simulink model "CM13_2024a_MachE_for_UA_HIL"  (R2024a)
settings: Solver=ode1  StartTime=0.0  StopTime=Inf  FixedStep=0.001  RelTol=1e-3  EnableMultiTasking=on
PreLoadFcn:
  | % if ~length(which('cmcmd')), cmenv; end
PostLoadFcn:
  | if any(exist('dsrtsu_mdlpostloadfcn', 'file') ~= 0), dsrtsu_mdlpostloadfcn('Execute', bdroot); end
InitFcn:
  | , if any(exist('rtifpga_mdlclblib', 'file') ~= 0), rtifpga_mdlclblib('Init', bdroot); end,
  | , if any(exist('dsmpb_private', 'file') ~= 0), dsmpb_private('dsmpb_mdlclblib', 'Init', bdroot); end,
values from neighbouring files (symbols this model uses):
  CoastDown =     [Run_Simulink.mat]
  limitedMCT =     [Run_Simulink.mat]
  MCT =     [Run_Simulink.mat]
  pMCT =     [Run_Simulink.mat]
  RealSimPara =     [Run_Simulink.mat]
  Ref_speed = [13 13.007895099 13.015778396 13.023649891 13.031509584 13.039357475 13.047193564 13.055017851 13.062830336 13.070631019 13.0784199 13.086196979 ... (2669 elements, 2669x1)]    [Ref_speed_and_time.mat]
  Ref_time = [0 0.01 0.02 0.03 0.04 0.05 0.06 0.07 0.08 0.09 0.1 0.11 ... (2669 elements, 2669x1)]    [Ref_speed_and_time.mat]
  US06 =     [Run_Simulink.mat]
undefined symbols (not defined in the file or in its folder): AccelCmd, ActTqLF_Nm_, ActTqLR_Nm_, ActTqRF_Nm_, ActTqRR_Nm_, BattChargeLimitMaxPwr, BattChargeLimitSocBpts, BattChargeLimitTbl, BattChrgCapcty, BattDischargeLimitSocBpts, BattDischargeLimitTbl, BattDischargeMaxPwr, BattNumCellsParallel, BattNumCellsSeries, BattOpenVoltCapBpts, BattOpenVoltTbl, BattResistSocBpts, BattResistTbl, BattResistTempBpts, BrakeMaxPrs, BrakeMaxTrq, ChassisDistCg2FrontAxle, ChassisDistCg2RearAxle, ChassisVehMass, CltchCmd, DecelCmd, DiffRatio, DiscIntNeverNeededParam, EnvGravCnst, EnvPrs, EnvTemp, FuelSpecificGrav, GearCmd, h, InitStates, lgSw, MtrEffSpdBpts, MtrEffTbl, MtrEffTrqBpts, MtrPwrMax, MtrTrqMax, planned_speed, planned_time, ref_speed, ref_time, rticanmm_blockfcn, rticanmm_initfcn, SteeringCmd, SupvsryCtrlRegenBrkCutOffTbl, SupvsryCtrlRegenSpdBpts, TestScnrioCycleNum, VEH
libraries: simulink x264, VSIGenLib x262, etargetslib x201, dsmpblib x161, CarMaker4SL x142, rtimmsu_dsrtlib x32, vehdynlibtire x24, autolibshared x19, vehdynlibsuspension x14, vehdynlibtirecommon x14, autolibutils x10, VsrLibWheel x8
(part 19 of 48)

== system CM13_2024a_MachE_for_UA_HIL/Vehicle Under Test3/Vehicle/Rototest and ORNL Interface/DummyPT ==
  WhlSpeedIn : Inport
  APPToTorque : Lookup_n-D  NumberOfTableDimensions=1  BreakpointsForDimension1=[0 100]  Table=[0 184]  InternalRulePriority=Speed  RndMeth=Simplest
  APPToTorque1 : Lookup_n-D  NumberOfTableDimensions=1  BreakpointsForDimension1=[0 100]  Table=[0 184]  InternalRulePriority=Speed  RndMeth=Simplest
  APP_pct : Constant  Value=0
  BPP_pct : Constant  Value=0
  FDR : Gain  Gain=3.18
  Flip : Gain  Gain=-1
  Gear : Product
  Memory : Memory
  NissanTrans : Lookup_n-D  NumberOfTableDimensions=1  BreakpointsForDimension1=[0 5 10 15 25 34 45 55]  Table=[5.25 3.03 1.95 1.46 1.22 1.00 0.81 0.67]  ExtrapMethod=Clip  InternalRulePriority=Speed  RndMeth=Simplest
  Sum : Sum  Inputs=++|
  WheelRadius : Gain  Gain=0.3235
  kph2mph : Gain  Gain=0.621
  mps2kph : Gain  Gain=3.6
  WheelTorqueOut : Outport
  wires:
  kph2mph/1 -> NissanTrans/1  "Speed_mph"
  APPToTorque/1 -> Sum/1  "APPTorque"
  mps2kph/1 -> kph2mph/1  "Speed_kph"
  BPP_pct/1 -> APPToTorque1/1
  NissanTrans/1 -> Gear/2  "Gear"
  Gear/1 -> FDR/1  "TransTorqueOut"
  APPToTorque1/1 -> Flip/1
  Flip/1 -> Sum/2  "BPPTorque"
  APP_pct/1 -> APPToTorque/1
  Sum/1 -> Gear/1  "TorqueTotal"
  WheelRadius/1 -> mps2kph/1  "Speed_mps"
  FDR/1 -> Memory/1  "WheelTorqueOut"
  WhlSpeedIn/1 -> WheelRadius/1
  Memory/1 -> WheelTorqueOut/1

== system CM13_2024a_MachE_for_UA_HIL/Vehicle Under Test3/Vehicle/Rototest and ORNL Interface/Format CM Powertrain Signals ==
  note: Can Bypass with my own brake model
  BrakingTorques : Inport
  RotoWheelSpd : Inport  Port=2
  AxlTrq : Inport  Port=3
  MaxRegen : Inport  Port=4
  Bus Creator1 : BusCreator  Inputs=42
  Bus Selector2 : BusSelector  OutputSignals=Brake IF Trq_WB FL,Brake IF Trq_WB FR,Brake IF Trq_WB RL,Brake IF Trq_WB RR
  BusCreator2 : BusCreator  Inputs=42
  Demux : Demux
  Demux1 : Demux  Outputs=42
      settings: DisplayOption=none
  Demux2 : Demux
  Discrete-Time Integrator{4..7} (4 alike) : DiscreteIntegrator  IntegratorMethod=Integration: Backward Euler  SampleTime=0.001  ICPrevOutput=DiscIntNeverNeededParam  ICPrevScaledInput=DiscIntNeverNeededParam
  Gain{5..8} (4 alike) : Gain  Gain=-1
  Ground{2..5} (4 alike) : Ground
  Ignition : Constant
  Memory{1..4} (4 alike) : Memory
  Operation Error : Constant  Value=4
  Operation State Driving : Constant  Value=4
  Product{1..4} (4 alike) : Product  RndMeth=Zero
  Saturation{1..4} (4 alike) : Saturate  UpperLimit=1  LowerLimit=-1
  Zero{1..5} (5 alike) : Constant  Value=0
  PowerTrainOutIdeal : Outport
  wires:
  Saturation4/1 -> Product4/2
  Demux1/3 -> BusCreator2/3  "PT IF OperationError"
  Demux1/2 -> BusCreator2/2  "PT IF OperationState"
  Demux1/40 -> BusCreator2/40  "PT IF WRR Trq_Supp2WC"
  Demux1/9 -> BusCreator2/9  "PT IF Trq_Supp2Bdy1B x"
  Discrete-Time Integrator6/1 -> Bus Creator1/29  "PT WRL rot"
  Demux1/1 -> BusCreator2/1  "PT IF Ignition"
  MaxRegen/1 -> Bus Creator1/28, Bus Creator1/21
  BusCreator2/1 -> PowerTrainOutIdeal/1
  Operation State Driving/1 -> Bus Creator1/2
  Gain8/1 -> Bus Creator1/38
  Demux1/16 -> BusCreator2/16  "PT IF WFL rotv"
  Demux1/21 -> BusCreator2/21  "PT IF WFL Trq_BrakeReg_max"
  Ground2/1 -> Bus Creator1/7
  Demux1/23 -> BusCreator2/23  "PT IF WFR rotv"
  Demux1/14 -> BusCreator2/14  "PT IF DL_iDiff_mean"
  Demux1/4 -> BusCreator2/4  "PT IF GearNo"
  Demux1/17 -> BusCreator2/17  "PT IF WFL Trq_B2W"
  Product3/1 -> Gain5/1
  Demux1/5 -> BusCreator2/5  "PT IF Engine_rotv"
  Demux1/11 -> BusCreator2/11  "PT IF Trq_Supp2Bdy1B z"
  Demux1/12 -> BusCreator2/12  "PT IF Trq_Supp2BdyEng x"
  Demux1/7 -> BusCreator2/7  "PT IF Trq_Supp2Bdy1 y"
  Discrete-Time Integrator5/1 -> Bus Creator1/22  "PT WFR rot"
  Demux1/42 -> BusCreator2/42  "PT IF WRR Trq_BrakeReg_max"
  Gain5/1 -> Bus Creator1/17
  Demux1/18 -> BusCreator2/18  "PT IF WFL Trq_Drive"
  Demux1/8 -> BusCreator2/8  "PT IF Trq_Supp2Bdy1 z"
  Demux1/38 -> BusCreator2/38  "PT IF WRR Trq_B2W"
  Memory4/1 -> Saturation4/1
  Demux1/10 -> BusCreator2/10  "PT IF Trq_Supp2Bdy1B y"
  Demux1/27 -> BusCreator2/27  "PT IF WFR Trq_BrakeReg"
  Demux1/24 -> BusCreator2/24  "PT IF WFR Trq_B2W"
  Demux1/25 -> BusCreator2/25  "PT IF WFR Trq_Drive"
  Demux1/26 -> BusCreator2/26  "PT IF WFR Trq_Supp2WC"
  Demux1/13 -> BusCreator2/13  "PT IF Trq_Supp2BdyEng y"
  Demux1/15 -> BusCreator2/15  "PT IF WFL rot"
  Bus Selector2/2 -> Product1/1  "<Brake IF Trq_WB FR>"
  Memory3/1 -> Saturation3/1
  Demux1/19 -> BusCreator2/19  "PT IF WFL Trq_Supp2WC"
  Demux1/22 -> BusCreator2/22  "PT IF WFR rot"
  Demux1/29 -> BusCreator2/29  "PT IF WRL rot"
  Demux1/33 -> BusCreator2/33  "PT IF WRL Trq_Supp2WC"
  Demux1/30 -> BusCreator2/30  "PT IF WRL rotv"
  Demux1/28 -> BusCreator2/28  "PT IF WFR Trq_BrakeReg_max"
  Demux1/35 -> BusCreator2/35  "PT IF WRL Trq_BrakeReg_max"
  Demux1/39 -> BusCreator2/39  "PT IF WRR Trq_Drive"
  Zero4/1 -> Bus Creator1/33, Bus Creator1/34, Bus Creator1/35
  Demux1/34 -> BusCreator2/34  "PT IF WRL Trq_BrakeReg"
  Demux1/37 -> BusCreator2/37  "PT IF WRR rotv"
  Demux1/31 -> BusCreator2/31  "PT IF WRL Trq_B2W"
  Demux1/32 -> BusCreator2/32  "PT IF WRL Trq_Drive"
  Demux1/36 -> BusCreator2/36  "PT IF WRR rot"
  Zero3/1 -> Bus Creator1/26, Bus Creator1/27
  Demux/4 -> Memory4/1, Discrete-Time Integrator7/1, Bus Creator1/37  "rotv RR"
  Zero2/1 -> Bus Creator1/19, Bus Creator1/20
  Zero1/1 -> Bus Creator1/5, Bus Creator1/4, Bus Creator1/12, Bus Creator1/14, Bus Creator1/13, Bus Creator1/11, Bus Creator1/10, Bus Creator1/9, Bus Creator1/8
  Demux1/20 -> BusCreator2/20  "PT IF WFL Trq_BrakeReg"
  Product2/1 -> Gain7/1
  Discrete-Time Integrator4/1 -> Bus Creator1/15  "PT WFL rot"
  Demux/2 -> Memory1/1, Discrete-Time Integrator5/1, Bus Creator1/23  "rotv FR"
  Discrete-Time Integrator7/1 -> Bus Creator1/36  "PtT WRR rot"
  Zero5/1 -> Bus Creator1/40, Bus Creator1/41, Bus Creator1/42
  Demux1/6 -> BusCreator2/6  "PT IF Trq_Supp2Bdy1 x"
  Demux1/41 -> BusCreator2/41  "PT IF WRR Trq_BrakeReg"
  BrakingTorques/1 -> Bus Selector2/1
  Operation Error/1 -> Bus Creator1/3
  Demux/3 -> Memory2/1, Discrete-Time Integrator6/1, Bus Creator1/30  "rotv RL"
  Memory1/1 -> Saturation1/1
  Ground4/1 -> Bus Creator1/6
  Bus Selector2/1 -> Product3/1  "<Brake IF Trq_WB FL>"
  Gain6/1 -> Bus Creator1/24
  Ignition/1 -> Bus Creator1/1  "PT Ignition"
  Memory2/1 -> Saturation2/1
  Saturation1/1 -> Product1/2
  Bus Selector2/3 -> Product2/1  "<Brake IF Trq_WB RL>"
  Gain7/1 -> Bus Creator1/31
  Demux/1 -> Memory3/1, Discrete-Time Integrator4/1, Bus Creator1/16  "rotv FL"
  Product4/1 -> Gain8/1
  Bus Creator1/1 -> Demux1/1
  Saturation2/1 -> Product2/2
  Product1/1 -> Gain6/1
  Bus Selector2/4 -> Product4/1  "<Brake IF Trq_WB RR>"
  Saturation3/1 -> Product3/2
  RotoWheelSpd/1 -> Demux/1
  AxlTrq/1 -> Demux2/1
  Demux2/1 -> Bus Creator1/18  "TrqDrv FL"
  Demux2/2 -> Bus Creator1/25  "TrqDrv FR"
  Demux2/3 -> Bus Creator1/32  "TrqDrv RL"
  Demux2/4 -> Bus Creator1/39  "TrqDrv RR"

== system CM13_2024a_MachE_for_UA_HIL/Vehicle Under Test3/Vehicle/Rototest and ORNL Interface/From Rototest ==
  Input : Inport
  Bus Creator : BusCreator  Inputs=30
  Bus Selector1 : BusSelector  OutputSignals=ActSpLF_rpm,ActSpRF_rpm,ActSpLR_rpm,ActSpRR_rpm
  Mux1 : Mux
  RotoTestEthRX : Subsystem  AncestorBlock=VSIGenLib/RotoTestEthRX
      mask Display:
      | color('white')
      | disp('RotTestEthTx')
      | port_label('output', 1, 'ID')
      | port_label('output', 2, 'ProtocolVer')
      | port_label('output', 3, 'ActTqLF (Nm)')
      | port_label('output', 4, 'RefRR_NmORrpm')
      | port_label('output', 5, 'ActTempLF (C)')
      | port_label('output', 6, 'ActTqRF (Nm)')
      | port_label('output', 7, 'ActSpRF (rpm)')
      | port_label('output', 8, 'ActTempRF (C)')
      | port_label('output', 9, 'ActTqLR (Nm)')
      | port_label('output', 10, 'ActSpLR (rpm)')
      | port_label('output', 11, 'ActTempLR (C)')
      | port_label('output', 12, 'ActTqRR (Nm)')
      | port_label('output', 13, 'ActSpRR (rpm)')
      | port_label('output', 14, 'ActTempRR (Nm)')
      | port_label('output', 15, 'RefLF (Nm)')
      | port_label('output', 16, 'RefRF (rpm)')
      | port_label('output', 17, 'RefLR (Nm)')
      | port_label('output', 18, 'RefRR (Nm)')
      | port_label('output', 19, 'UnitsStatusLF (enum)')
      | port_label('output', 20, 'UnitsStatusRF (enum)')
      | port_label('output', 21, 'UnitsStatusLR (enum)')
      | port_label('output', 22, 'UnitsStatusRR (enum)')
      | port_label('output', 23, 'WatchdogCnt (int)')
      | port_label('output', 24, 'FaultActive (enum)')
      | port_label('output', 25, 'WarningsActive (enum)')
      | port_label('output', 26, 'SpTqRR (enum)')
      | port_label('output', 27, 'SpTqLR (enum)')
      | port_label('output', 28, 'SpTqRF (enum)')
      | port_label('output', 29, 'SpTqLF (enum)')
      | port_label('output', 30, 'SystemActive (bool)')
  SpdAct : Outport
  AxlTrq : Outport  Port=2
  wires:
  RotoTestEthRX/8(ActTempRF_C) -> Bus Creator/8
  RotoTestEthRX/23(WatchdogCnt) -> Bus Creator/23
  RotoTestEthRX/18(RefRR_Nm) -> Bus Creator/18
  Mux1/1 -> SpdAct/1
  RotoTestEthRX/19(UnitsStatusLF) -> Bus Creator/19
  RotoTestEthRX/4(ActSpLF_rpm) -> Bus Creator/4
  Bus Creator/1 -> AxlTrq/1, Bus Selector1/1
  Bus Selector1/4 -> Mux1/4  "<ActSpRR_rpm>"
  RotoTestEthRX/24(FaultActive) -> Bus Creator/24
  RotoTestEthRX/22(UnitsStatusRR) -> Bus Creator/22
  Bus Selector1/3 -> Mux1/3  "<ActSpLR_rpm>"
  RotoTestEthRX/25(WarningsActive) -> Bus Creator/25
  Bus Selector1/1 -> Mux1/1  "<ActSpLF_rpm>"
  Bus Selector1/2 -> Mux1/2  "<ActSpRF_rpm>"
  RotoTestEthRX/5(ActTempLF_C) -> Bus Creator/5
  RotoTestEthRX/30(SystemActive) -> Bus Creator/30
  RotoTestEthRX/20(UnitsStatusRF) -> Bus Creator/20
  RotoTestEthRX/15(RefLF_Nm) -> Bus Creator/15
  RotoTestEthRX/16(RefRF_rpm) -> Bus Creator/16
  RotoTestEthRX/17(RefLR_Nm) -> Bus Creator/17
  RotoTestEthRX/2(ProtocolVer) -> Bus Creator/2
  RotoTestEthRX/7(ActSpRF_rpm) -> Bus Creator/7
  RotoTestEthRX/21(UnitsStatusLR) -> Bus Creator/21
  RotoTestEthRX/11(ActTempLR_C) -> Bus Creator/11
  RotoTestEthRX/1(ID) -> Bus Creator/1
  RotoTestEthRX/28(SpTqRF) -> Bus Creator/28
  RotoTestEthRX/29(SpTqLF) -> Bus Creator/29
  RotoTestEthRX/27(SpTqLR) -> Bus Creator/27
  RotoTestEthRX/26(SpTqRR) -> Bus Creator/26
  RotoTestEthRX/14(ActTempRR_Nm) -> Bus Creator/14
  RotoTestEthRX/3(ActTqLF_Nm) -> Bus Creator/3
  RotoTestEthRX/6(ActTqRF_Nm_) -> Bus Creator/6
  RotoTestEthRX/9(ActTqLR_Nm) -> Bus Creator/9
  RotoTestEthRX/13(ActSpRR_rpm) -> Bus Creator/13
  RotoTestEthRX/10(ActSpLR_rpm) -> Bus Creator/10
  RotoTestEthRX/12(ActTqRR_Nm) -> Bus Creator/12
  Input/1 -> RotoTestEthRX/1(Input)

== system CM13_2024a_MachE_for_UA_HIL/Vehicle Under Test3/Vehicle/Rototest and ORNL Interface/Get Wheel Spd Cmd Based on Wheel Dynamics ==
  BrakingTorques : Inport
  Trq_T2W : Inport  Port=2
  AxlTrq : Inport  Port=3
  MaxRegen : Inport  Port=4
  FxIn : Inport  Port=5
  Saturation : Saturate  UpperLimit=100  LowerLimit=0
  Saturation1 : Saturate  UpperLimit=300  LowerLimit=-300
  Scope : Scope
  WheelSpdCmd : Subsystem
  Whl Dynamics & Format CM Powertrain Signal : Subsystem
  WhlSpdCmd : Outport
  wires:
  Whl Dynamics & Format CM Powertrain Signal/1(PowerTrainOutIdeal) -> WheelSpdCmd/1(In1)
  BrakingTorques/1 -> Whl Dynamics & Format CM Powertrain Signal/1(BrakingTorques)
  Trq_T2W/1 -> Whl Dynamics & Format CM Powertrain Signal/2(Trq_T2W)
  MaxRegen/1 -> Whl Dynamics & Format CM Powertrain Signal/4(MaxRegen)
  AxlTrq/1 -> Whl Dynamics & Format CM Powertrain Signal/3(AxlTrq)
  FxIn/1 -> Whl Dynamics & Format CM Powertrain Signal/5(FxIn)
  [SimOmega] -> Scope/1, Saturation/1
  Saturation/1 -> WhlSpdCmd/1

== system CM13_2024a_MachE_for_UA_HIL/Vehicle Under Test3/Vehicle/Rototest and ORNL Interface/RotoTrqPreprocess ==
  AxleTrqRaw : Inport
  Bus Selector1 : BusSelector  OutputSignals=ActTqLF_Nm_,ActTqRF_Nm_,ActTqLR_Nm_,ActTqRR_Nm_
  Compare To Constant : simulink/Logic and Bit Operations/Compare To Constant  relop=>=  const=-15  OutDataTypeStr=boolean
  Compare To Constant1 : simulink/Logic and Bit Operations/Compare To Constant  relop=<=  const=0  OutDataTypeStr=boolean
  Data Type Conversion{1..4} (4 alike) : DataTypeConversion  OutDataTypeStr=double  SaturateOnIntegerOverflow=off  RndMeth=Floor
  FirstOrderFilterTau{,1..3} (4 alike) : VSIGenLib/FirstOrderFilterTau  SystemSampleTime=-1  VariantActivationTime=update diagram  AllowFlexibleInterface=on  Latency=0  AutoFrameSizeCalculation=off
  Ground : Ground
  Logical Operator : Logic  AllPortsSameDT=off  OutDataTypeStr=boolean
  ManualTrq_Nm : Constant  Value=0
  Mux : Mux
  Mux1 : Mux
  SatTrq : Saturate  UpperLimit=1000  LowerLimit=-1000
  Tau : Constant  Value=0.01
  TorqueIn : Switch  Criteria=u2 > Threshold  SaturateOnIntegerOverflow=off  InputSameDT=off
  "TorqueIn " : Switch  Criteria=u2 > Threshold  SaturateOnIntegerOverflow=off  InputSameDT=off
  AxleTrqRoto : Outport
  AxleTrqVeh : Outport  Port=2
  wires:
  Mux/1 -> AxleTrqRoto/1, TorqueIn/1
  ManualTrq_Nm/1 -> Mux1/4, Mux1/3, Mux1/2, Mux1/1
  Tau/1 -> FirstOrderFilterTau/2, FirstOrderFilterTau1/2, FirstOrderFilterTau2/2, FirstOrderFilterTau3/2
  Ground/1 -> "TorqueIn "/1
  Logical Operator/1 -> "TorqueIn "/2
  Data Type Conversion4/1 -> Mux/4  "RR"
  Data Type Conversion3/1 -> Mux/3  "LR"
  Mux1/1 -> TorqueIn/3
  [Switch] -> TorqueIn/2
  Bus Selector1/4 -> FirstOrderFilterTau3/1  "<ActTqRR_Nm_>"
  Compare To Constant/1 -> Logical Operator/1
  Bus Selector1/3 -> FirstOrderFilterTau2/1  "<ActTqLR_Nm_>"
  Bus Selector1/2 -> FirstOrderFilterTau1/1  "<ActTqRF_Nm_>"
  TorqueIn/1 -> SatTrq/1
  "TorqueIn "/1 -> AxleTrqVeh/1  "Trq"
  FirstOrderFilterTau1/1 -> Data Type Conversion2/1
  Data Type Conversion2/1 -> Mux/2  "RF"
  AxleTrqRaw/1 -> Bus Selector1/1
  FirstOrderFilterTau/1 -> Data Type Conversion1/1
  FirstOrderFilterTau3/1 -> Data Type Conversion4/1
  Bus Selector1/1 -> FirstOrderFilterTau/1  "<ActTqLF_Nm_>"
  Compare To Constant1/1 -> Logical Operator/2
  SatTrq/1 -> "TorqueIn "/3, Compare To Constant1/1, Compare To Constant/1
  FirstOrderFilterTau2/1 -> Data Type Conversion3/1
  Data Type Conversion1/1 -> Mux/1  "LF"

== system CM13_2024a_MachE_for_UA_HIL/Vehicle Under Test3/Vehicle/Rototest and ORNL Interface/Subsystem2 ==
  AxlTorq : Inport
  BusCreator1 : BusCreator  Inputs=16
  BusCreator2 : BusCreator  Inputs=16
  Constant : Constant  Value=0
  Constant1 : Constant  Value=0
  Demux : Demux  Outputs=16
      settings: DisplayOption=none
  Terminator : Terminator
  Zero1 : Constant  Value=0
  Zero2 : Constant  Value=0
  Zero5 : Constant  Value=0
  BrakeUpd : Outport
  wires:
  Demux/9 -> BusCreator1/9  "Brake IF Trq_Reg_trg FL"
  Demux/6 -> BusCreator1/6  "Brake IF Trq_PB FR"
  Constant1/1 -> BusCreator2/1, BusCreator2/2  "Brake IF Trq_WB FL"
  Demux/14 -> BusCreator1/14  "Brake IF Trq_DriveSrc_trg d1"
  Zero2/1 -> BusCreator2/16, BusCreator2/15, BusCreator2/14, BusCreator2/13  "Brake IF Trq_DriveSrc_trg d3"
  Demux/11 -> BusCreator1/11  "Brake IF Trq_Reg_trg RL"
  Demux/15 -> BusCreator1/15  "Brake IF Trq_DriveSrc_trg d2"
  Demux/2 -> BusCreator1/2  "Brake IF Trq_WB FR"
  Demux/16 -> BusCreator1/16  "Brake IF Trq_DriveSrc_trg d3"
  Zero1/1 -> BusCreator2/12, BusCreator2/11, BusCreator2/10, BusCreator2/9  "Brake IF Trq_Reg_trg RR"
  Demux/4 -> BusCreator1/4  "Brake IF Trq_WB RR"
  Demux/3 -> BusCreator1/3  "Brake IF Trq_WB RL"
  Constant/1 -> BusCreator2/4, BusCreator2/3  "Brake IF Trq_WB RL"
  BusCreator1/1 -> BrakeUpd/1
  Demux/1 -> BusCreator1/1  "Brake IF Trq_WB FL"
  Demux/8 -> BusCreator1/8  "Brake IF Trq_PB RR"
  Demux/10 -> BusCreator1/10  "Brake IF Trq_Reg_trg FR"
  BusCreator2/1 -> Demux/1
  Demux/13 -> BusCreator1/13  "Brake IF Trq_DriveSrc_trg d0"
  Demux/5 -> BusCreator1/5  "Brake IF Trq_PB FL"
  Demux/7 -> BusCreator1/7  "Brake IF Trq_PB RL"
  Zero5/1 -> BusCreator2/8, BusCreator2/7, BusCreator2/6, BusCreator2/5  "Brake IF Trq_PB RR"
  Demux/12 -> BusCreator1/12  "Brake IF Trq_Reg_trg RR"
  AxlTorq/1 -> Terminator/1

== system CM13_2024a_MachE_for_UA_HIL/Vehicle Under Test3/Vehicle/Rototest and ORNL Interface/To Rototest with Band-Aid ==
  note: Torque Model: Low speed
      | Speed Model: Normal speed
  note: OutMode = 0 is Torque
      | OutMode = 1 is Speed
  note: Switch = 0 Overides
      | Switch = 1 Model
  SpeedCmd_rps : Inport
  AxleTrq_roto_Nm : Inport  Port=2
  BRAKE_PRESSED : Inport  Port=3
  Vehicle_Speed_kph : Inport  Port=4
  Band-Aid : Subsystem
  Demux : Demux
  Demux1 : Demux
  Demux2 : Demux
  Logging : Subsystem  Commented=on
  MasterSw : Constant  Value=0
  Mode Override : Subsystem
  ModeOut : Switch  Criteria=u2 > Threshold  SaturateOnIntegerOverflow=off  InputSameDT=off
  ModeSwitch : MultiPortSwitch  DataPortOrder=Zero-based contiguous  Inputs=2  zeroidx=on  SaturateOnIntegerOverflow=off  InputSameDT=off
  Mux2 : Mux
  Mux4 : Mux
  Mux5 : Mux
  RateLimSpd : RateLimiter  RisingSlewLimit=500  FallingSlewLimit=-500  SampleTimeMode=inherited
  RotoTestEthTx : Subsystem  AncestorBlock=VSIGenLib/RotoTestEthTx
      mask Display:
      | color('white')
      | disp('RotTestEthTx')
      | port_label('input', 1, 'RefLF_NmORrpm')
      | port_label('input', 2, 'RefRF_NmORrpm')
      | port_label('input', 3, 'RefLR_NmORrpm')
      | port_label('input', 4, 'RefRR_NmORrpm')
      | port_label('input', 5, 'SqTrRR')
      | port_label('input', 6, 'SqTrLR')
      | port_label('input', 7, 'SqTrRF')
      | port_label('input', 8, 'SqTrLF')
      | port_label('input', 9, 'SystemActive')
      | port_label('output', 1, 'Status (bool)')
      | port_label('output', 2, 'Sent Bytes (int)')
  SatSpd : Saturate  UpperLimit=500  LowerLimit=0
  Scope : Scope
  SpeedOut : Switch  Criteria=u2 > Threshold  SaturateOnIntegerOverflow=off  InputSameDT=off
  SystemActive : Constant  Value=0  OutDataTypeStr=uint8
  Transfer Fcn{,1..3} (4 alike) : TransferFcn  Denominator=[0.02 1]
  TrqSpd Override : Subsystem
  ZeroTorque : Constant  Value=0  OutDataTypeStr=uint8
  rads2rpm : Gain  Gain=9.5492965964254
  Out1 : Outport
  tag scope: Switch=global
  wires:
  Mux4/1 -> ModeSwitch/2
  Demux/3 -> Mux2/3  "LRIn"
  Demux1/4 -> Transfer Fcn3/1
  Demux/2 -> Mux2/2  "RFIn"
  MasterSw/1 -> [Switch]
  TrqSpd Override/1(Ovr) -> SpeedOut/3
  ZeroTorque/1 -> Mux4/2, Mux4/3, Mux4/4, Mux4/1
  Demux/1 -> Mux2/1  "LFIn"
  SpeedOut/1 -> RateLimSpd/1
  RateLimSpd/1 -> SatSpd/1
  rads2rpm/1 -> Demux/1
  ModeSwitch/1 -> Scope/1, Demux1/1
  Demux/4 -> Mux2/4  "RRIn"
  Band-Aid/1(OutMode) -> Mux5/4, Mux5/3, Mux5/2, Mux5/1, ModeSwitch/1
  ModeOut/1 -> Demux2/1
  [Switch] -> SpeedOut/2
  SatSpd/1 -> ModeSwitch/3  "Spd"
  [Switch] -> ModeOut/2
  Mux5/1 -> ModeOut/1
  Demux2/1 -> RotoTestEthTx/5(SpTqRR)
  Demux1/3 -> Transfer Fcn2/1
  Demux2/3 -> RotoTestEthTx/7(SpTqRF)
  Demux2/2 -> RotoTestEthTx/6(SpTqLR)
  SystemActive/1 -> RotoTestEthTx/9(SystemActive)
  RotoTestEthTx/1(Output) -> Out1/1  "ByteSend"
  Demux1/1 -> Transfer Fcn/1
  Demux1/2 -> Transfer Fcn1/1
  Demux2/4 -> RotoTestEthTx/8(SpTqLF)
  SpeedCmd_rps/1 -> rads2rpm/1
  Mode Override/1(Ovr) -> ModeOut/3
  AxleTrq_roto_Nm/1 -> Band-Aid/2(InTrq_Nm)
  Mux2/1 -> Band-Aid/1(InSpd_rpm)
  Band-Aid/2(OutSpd_rpm) -> SpeedOut/1
  BRAKE_PRESSED/1 -> Band-Aid/3(BRAKE_PRESSED)
  Vehicle_Speed_kph/1 -> Band-Aid/4(VehSpd_kph)
  Transfer Fcn/1 -> RotoTestEthTx/1(RefLF_NmORrpm)
  Transfer Fcn1/1 -> RotoTestEthTx/2(RefRF_NmORrpm)
  Transfer Fcn2/1 -> RotoTestEthTx/3(RefLR_NmORrpm)
  Transfer Fcn3/1 -> RotoTestEthTx/4(RefRR_NmORrpm)

== system CM13_2024a_MachE_for_UA_HIL/Vehicle Under Test3/Vehicle/Vehicle Dynamics/Vehicle 14DOF ==
  Env : Inport
  SupvsryCtrl : Inport  Port=2
  AxlTrq : Inport  Port=3
  AxT{,1..7} (8 alike) : Scope
  Brake Pressure : Subsystem
  BrkPrs : Scope
  Bus Creator : BusCreator  Inputs=5
  Bus Creator1 : BusCreator  Inputs=ActTqLF_Nm_,ActTqRF_Nm_,ActTqLR_Nm_,ActTqRR_Nm_
  Bus Creator2 : BusCreator  Inputs=Car Trq_T2WFL,Car Trq_T2WFR,Car Trq_T2WRL,Car Trq_T2WRR
  Bus Selector : BusSelector  OutputSignals=SteeringCmd
  Bus Selector1 : BusSelector  OutputSignals=BrkCmd
  Bus Selector2 : BusSelector  OutputSignals=WindVel,GndBus.z,GndBus.mu
  Bus Selector3 : BusSelector  OutputSignals=G_FL_z,G_FR_z,G_RL_z,G_RR_z
  Bus Selector4 : BusSelector  OutputSignals=mu_FL,mu_FR,mu_RL,mu_RR
  Bus Selector5 : BusSelector  OutputSignals=TireFrame.My
  Bus Selector6 : BusSelector  OutputSignals=VehSpd
  Bus Selector7 : BusSelector  OutputSignals=TireFrame.Fx
  Bus Selector8 : BusSelector  OutputSignals=TireFrame.Omega
  Demux : Demux
  Demux1 : Demux
  Demux2 : Demux
  Mux : Mux
  Scope : Scope
  Scope1 : Scope
  Scope2 : Scope
  Steering : Subsystem
  Subsystem1 : Subsystem
  Subsystem4 : Subsystem  Commented=on
  Suspension : Subsystem  Variant=on  VariantControlMode=label  LabelModeActiveChoice=3
      mask Display:
      | switch str2num(get_param(gcb,'ActiveVariant'))
      |     case 1
      |         image('suspdw.png');
      |     case 2
      |         image([imread('suspindmap.png');imread('suspsamap.png')]);
      |     case 3
      |          image([imread('suspmacp.png');imread('suspsacoil.png')]);
      |     case 4
      |          image('suspmacp.png');
      |     case 5
      |          image('suspindmap.png');
      | end
  To Workspace2 : ToWorkspace  VariableName=TiTrq  SampleTime=-1
      settings: Save2DSignal=2-D array (concatenate along first dimension)
  To Workspace3 : ToWorkspace  VariableName=AxlTrq  SampleTime=-1
      settings: Save2DSignal=2-D array (concatenate along first dimension)
  To Workspace4 : ToWorkspace  VariableName=Fx  SampleTime=-1
      settings: Save2DSignal=2-D array (concatenate along first dimension)
  To Workspace5 : ToWorkspace  VariableName=Speed  SampleTime=-1
      settings: Save2DSignal=2-D array (concatenate along first dimension)
  To Workspace6 : ToWorkspace  VariableName=Omega  SampleTime=-1
      settings: Save2DSignal=2-D array (concatenate along first dimension)
  Transfer Fcn{,9..11} (4 alike) : TransferFcn  Denominator=[0.2 1]
  Transfer Fcn{1..4} (4 alike) : TransferFcn  Denominator=[0.1 1]
  Transfer Fcn{5..8} (4 alike) : TransferFcn  Denominator=[0.01 1]
  Vector Concatenate : Concatenate  NumInputs=4
  Vector Concatenate1 : Concatenate  NumInputs=4
  Vehicle : Subsystem
      mask Display: image('6dofcar.png');
  Vehicle Routing : Subsystem  Commented=on
  Vehicle Routing1 : Subsystem
  Wheel Routing : Subsystem  Commented=on
  Wheel Routing1 : Subsystem
  Wheels and Tires : Subsystem
      mask Display: image('wheel3dof.png')
  Whl : Outport
  Chassis : Outport  Port=2
  RototestInput : Outport  Port=3
  tag scope: vehSpeedSim=global
  wires:
  Wheels and Tires/1(Wheels) -> Bus Selector7/1, Bus Selector5/1, Suspension/3(Wheel), Bus Selector8/1, Wheel Routing1/2(Wheel)  "Wheels"
  Vehicle/1(VehFdbk) -> Vehicle Routing1/1(Veh), Wheel Routing1/1(Info), Suspension/2(Vehicle)  "Veh"
  Suspension/1(Suspension) -> Vehicle/1(Suspension), Wheels and Tires/1(Suspension)  "Susp"
  Bus Selector2/1 -> Scope/1, Vehicle/2(Wind)  "<WindVel>"
  Steering/1(WhlAng) -> AxT7/1, Suspension/1(Steering)
  Bus Selector/1 -> Steering/1(SteeringCmd)  "<SteeringCmd>"
  SupvsryCtrl/1 -> Bus Selector/1, Bus Selector1/1
  Bus Selector1/1 -> Brake Pressure/1(BrkReq)  "<BrkCmd>"
  Env/1 -> Bus Selector2/1
  Subsystem1/2(Wheels) -> Whl/1
  AxlTrq/1 -> Demux1/1, AxT2/1, Wheels and Tires/2(Axle Torque)
  Bus Selector2/2 -> Bus Selector3/1  "<z>"
  Bus Selector3/1 -> Scope1/1, Vector Concatenate/1  "<G_FL_z>"
  Bus Selector3/2 -> Vector Concatenate/2  "<G_FR_z>"
  Bus Selector3/3 -> Vector Concatenate/3  "<G_RL_z>"
  Bus Selector3/4 -> Vector Concatenate/4  "<G_RR_z>"
  Vector Concatenate/1 -> Wheels and Tires/4(Ground Input)
  Bus Selector4/4 -> Vector Concatenate1/4  "<mu_RR>"
  Bus Selector2/3 -> Bus Selector4/1  "<mu>"
  Bus Selector4/3 -> Vector Concatenate1/3  "<mu_RL>"
  Bus Selector4/2 -> Vector Concatenate1/2  "<mu_FR>"
  Bus Selector4/1 -> Scope2/1, Vector Concatenate1/1  "<mu_FL>"
  Vector Concatenate1/1 -> Wheels and Tires/5(Friction)
  Bus Selector6/1 -> AxT6/1, [vehSpeedSim], To Workspace5/1, Bus Creator/4  "<VehSpd>"
  Brake Pressure/1(BrakePrs) -> BrkPrs/1, Bus Creator/3, Wheels and Tires/3(Brake Press)  "BrakePressed_flag"
  Bus Creator1/1 -> To Workspace3/1, Bus Creator/2  "AxleTrq"
  Bus Creator2/1 -> Bus Creator/1, AxT3/1, To Workspace2/1  "CarTrqT2W"
  Bus Selector5/1 -> Demux/1, AxT/1  "<My>"
  Subsystem1/1(Chassis) -> Bus Selector6/1, Chassis/1
  Bus Selector7/1 -> Demux2/1, AxT1/1, To Workspace4/1  "<Fx>"
  Bus Selector8/1 -> AxT5/1, To Workspace6/1  "<Omega>"
  Bus Creator/1 -> RototestInput/1
  Transfer Fcn5/1 -> Bus Creator1/1  "ActTqLF_Nm_"
  Demux1/3 -> Transfer Fcn7/1  "ActTqLR_Nm_"
  Transfer Fcn8/1 -> Bus Creator1/4  "ActTqRR_Nm_"
  Demux1/2 -> Transfer Fcn6/1  "ActTqRF_Nm_"
  Transfer Fcn6/1 -> Bus Creator1/2  "ActTqRF_Nm_"
  Demux1/1 -> Transfer Fcn5/1  "ActTqLF_Nm_"
  Transfer Fcn7/1 -> Bus Creator1/3  "ActTqLR_Nm_"
  Demux1/4 -> Transfer Fcn8/1  "ActTqRR_Nm_"
  Demux2/3 -> Transfer Fcn10/1
  Transfer Fcn10/1 -> Mux/3
  Demux2/2 -> Transfer Fcn9/1
  Transfer Fcn9/1 -> Mux/2
  Demux2/4 -> Transfer Fcn11/1
  Transfer Fcn/1 -> Mux/1
  Demux2/1 -> Transfer Fcn/1
  Transfer Fcn11/1 -> Mux/4
  Mux/1 -> Bus Creator/5, AxT4/1  "Fx"
  Transfer Fcn3/1 -> Bus Creator2/1  "Car Trq_T2WFL"
  Demux/3 -> Transfer Fcn2/1  "Car Trq_T2WRL"
  Transfer Fcn1/1 -> Bus Creator2/2  "Car Trq_T2WFR"
  Demux/2 -> Transfer Fcn1/1  "Car Trq_T2WFR"
  Demux/1 -> Transfer Fcn3/1  "Car Trq_T2WFL"
  Demux/4 -> Transfer Fcn4/1  "Car Trq_T2WRR"
  Transfer Fcn4/1 -> Bus Creator2/4  "Car Trq_T2WRR"
  Transfer Fcn2/1 -> Bus Creator2/3  "Car Trq_T2WRL"
  Vehicle Routing/2(CgXYZ) -> Subsystem4/2(CgXYZ)
  Vehicle Routing/5(pqr) -> Subsystem4/5(pqr)
  Vehicle Routing/1(Cgxyzdot) -> Subsystem4/1(Cgxyzdot)
  Wheel Routing/2(Kappa) -> Subsystem4/11(Kappa)
  Wheel Routing/6(ZWheel) -> Subsystem4/15(dzWheel)
  Wheel Routing/5(YWheel) -> Subsystem4/14(YWheel)
  Wheel Routing/3(Alpha) -> Subsystem4/12(Alpha)
  Wheel Routing/1(Omega) -> Subsystem4/10(Omega)
  Wheel Routing/4(XWheel) -> Subsystem4/13(XWheel)
  Vehicle Routing/7(Beta) -> Subsystem4/7(Beta)
  Vehicle Routing/4(angles) -> Subsystem4/4(angles)
  Vehicle Routing/9(GeomXYZdot) -> Subsystem4/9(GeomXYZdot)
  Vehicle Routing/3(CgXYZdot) -> Subsystem4/3(CgXYZdot)
  Vehicle Routing/6(Cgaxyz) -> Subsystem4/6(Cgaxyz)
  Vehicle Routing/8(GeomXYZ) -> Subsystem4/8(GeomXYZ)
  Vehicle Routing1/10(Cgxyzdotdot) -> Subsystem1/10(Cgxyzdotdot)
  Wheel Routing1/6(ZWheel) -> Subsystem1/16(dzWheel)
  Wheel Routing1/5(YWheel) -> Subsystem1/15(YWheel)
  Wheel Routing1/2(Kappa) -> Subsystem1/12(Kappa)
  Wheel Routing1/4(XWheel) -> Subsystem1/14(XWheel)
  Wheel Routing1/3(Alpha) -> Subsystem1/13(Alpha)
  Wheel Routing1/1(Omega) -> Subsystem1/11(Omega)
  Vehicle Routing1/6(Cgaxyz) -> Subsystem1/6(Cgaxyz)
  Vehicle Routing1/2(CgXYZ) -> Subsystem1/2(CgXYZ)
  Vehicle Routing1/7(Beta) -> Subsystem1/7(Beta)
  Vehicle Routing1/3(CgXYZdot) -> Subsystem1/3(CgXYZdot)
  Vehicle Routing1/4(angles) -> Subsystem1/4(angles)
  Vehicle Routing1/5(pqr) -> Subsystem1/5(pqr)
  Vehicle Routing1/1(Cgxyzdot) -> Subsystem1/1(Cgxyzdot)
  Vehicle Routing1/8(GeomXYZ) -> Subsystem1/8(GeomXYZ)
  Vehicle Routing1/9(GeomXYZdot) -> Subsystem1/9(GeomXYZdot)

== system CM13_2024a_MachE_for_UA_HIL/Vehicle Under Test3/Vehicle/Vehicle Dynamics/Vehicle 7DOF ==
  Env : Inport
  SupvsryCtrl : Inport  Port=2
  AxlTrq : Inport  Port=3
  Brake Pressure : Subsystem
  Bus Creator : BusCreator  Inputs=5
  Bus Selector : BusSelector  OutputSignals=SteeringCmd
  Bus Selector1 : BusSelector  OutputSignals=BrkCmd
  Bus Selector10 : BusSelector  OutputSignals=InertFrm.Geom.Disp.X,InertFrm.Geom.Disp.Y,InertFrm.Geom.Disp.Z  OutputAsBus=on
  Bus Selector11 : BusSelector  OutputSignals=InertFrm.Geom.Vel.Xdot,InertFrm.Geom.Vel.Ydot,InertFrm.Geom.Vel.Zdot  OutputAsBus=on
  Bus Selector12 : BusSelector  OutputSignals=BdyFrm.Geom.Ang.Beta
  Bus Selector13 : BusSelector  OutputSignals=BdyFrm.Cg.Vel.xdot,BdyFrm.Cg.Vel.ydot,BdyFrm.Cg.Vel.zdot  OutputAsBus=on
  Bus Selector2 : BusSelector  OutputSignals=WindVel,GndBus.z,GndBus.mu
  Bus Selector3 : BusSelector  OutputSignals=G_FL_z,G_FR_z,G_RL_z,G_RR_z
  Bus Selector4 : BusSelector  OutputSignals=mu_FL,mu_FR,mu_RL,mu_RR
  Bus Selector5 : BusSelector  OutputSignals=InertFrm.Cg.Disp.X,InertFrm.Cg.Disp.Y,InertFrm.Cg.Disp.Z  OutputAsBus=on
  Bus Selector6 : BusSelector  OutputSignals=InertFrm.Cg.Vel.Xdot,InertFrm.Cg.Vel.Ydot,InertFrm.Cg.Vel.Zdot  OutputAsBus=on
  Bus Selector7 : BusSelector  OutputSignals=BdyFrm.Cg.Acc.ax,BdyFrm.Cg.Acc.ay,BdyFrm.Cg.Acc.az  OutputAsBus=on
  Bus Selector8 : BusSelector  OutputSignals=InertFrm.Cg.Ang.phi,InertFrm.Cg.Ang.theta,InertFrm.Cg.Ang.psi  OutputAsBus=on
  Bus Selector9 : BusSelector  OutputSignals=BdyFrm.Cg.AngVel.p,BdyFrm.Cg.AngVel.q,BdyFrm.Cg.AngVel.r  OutputAsBus=on
  Bus to Vector{,1..7} (8 alike) : BusToVector
  Constant : Constant  Value=0
  For 3D Visualization : MATLAB Function  TreatAsAtomicUnit=on  mask{trackW=1.9, wheelB=ChassisDistCg2FrontAxle+ChassisDistCg2RearAxle}
      mask prompts: trackW "Vehicle track width, trackW [m]:"; wheelB "Vehicle wheelbase, wheelB [m]:"
      mask help: This block converts wheel ground height information into estimates of vehicle pitch, roll angles and vertical height in order to help in the visualization 3DOF based simulations with changes in terrain. Note that the resulting signals are only used as a visualization aid and do not account for the physical affects of the vehicle interacting with variable terrain or changes in orientation.
  Longitudinal Wheels 4DOF : Subsystem  VariantControl=1
      settings: AttributesFormatString=%<wheelMode>
  RototestDummy : Subsystem
  Steering : Subsystem
  Subsystem4 : Subsystem
  Terminator : Terminator
  Vector Concatenate : Concatenate  NumInputs=4
  Vector Concatenate1 : Concatenate  NumInputs=4
  Vector Concatenate2 : Concatenate  NumInputs=4
  Vehicle Body 3DOF External Longitudinal Wheels : Subsystem  Variant=on  VariantControlMode=label  VariantControl=Variant1  LabelModeActiveChoice=1
      settings: AttributesFormatString=%<trackMode>
  Whl : Outport
  Chassis : Outport  Port=2
  RototestInput : Outport  Port=3
  wires:
  Bus Selector2/1 -> Vehicle Body 3DOF External Longitudinal Wheels/4(WindXYZ)  "<WindVel>"
  Bus Selector/1 -> Steering/1(SteeringCmd)  "<SteeringCmd>"
  SupvsryCtrl/1 -> Bus Selector/1, Bus Selector1/1
  Bus Selector1/1 -> Brake Pressure/1(BrkReq)  "<BrkCmd>"
  Env/1 -> Bus Selector2/1
  Subsystem4/2(Wheels) -> Whl/1
  Subsystem4/1(Chassis) -> Chassis/1
  Bus Selector2/2 -> Bus Selector3/1  "<z>"
  Bus Selector3/1 -> Vector Concatenate/1  "<G_FL_z>"
  Bus Selector3/2 -> Vector Concatenate/2  "<G_FR_z>"
  Bus Selector3/3 -> Vector Concatenate/3  "<G_RL_z>"
  Bus Selector3/4 -> Vector Concatenate/4  "<G_RR_z>"
  Bus Selector4/4 -> Vector Concatenate1/4  "<mu_RR>"
  Bus Selector2/3 -> Bus Selector4/1  "<mu>"
  Bus Selector4/3 -> Vector Concatenate1/3  "<mu_RL>"
  Bus Selector4/2 -> Vector Concatenate1/2  "<mu_FR>"
  Bus Selector4/1 -> Vector Concatenate1/1  "<mu_FL>"
  Vector Concatenate2/1 -> Terminator/1
  Constant/1 -> Vector Concatenate2/4, Vector Concatenate2/3, Vector Concatenate2/2, Vector Concatenate2/1
  Bus to Vector2/1 -> Subsystem4/6(Cgaxyz)  "Cgaxyz"
  Bus Selector8/1 -> Bus to Vector3/1
  Bus to Vector5/1 -> For 3D Visualization/2(GemoXYZIn)
  Bus Selector12/1 -> Subsystem4/7(Beta)  "<Beta>"
  Bus Selector5/1 -> Bus to Vector/1
  For 3D Visualization/1(angles) -> Subsystem4/4(angles)  "angles"
  For 3D Visualization/2(GeomXYZ) -> Subsystem4/8(GeomXYZ)  "GeomXYZ"
  Bus to Vector6/1 -> Subsystem4/9(GeomXYZdot)  "GeomXYZdot"
  Bus Selector13/1 -> Bus to Vector7/1
  Bus to Vector7/1 -> Subsystem4/1(Cgxyzdot)  "Cgxyzdot"
  Bus Selector10/1 -> Bus to Vector5/1
  Longitudinal Wheels 4DOF/1(FrntAxlF) -> Vehicle Body 3DOF External Longitudinal Wheels/2("FwF ")
  Bus Selector11/1 -> Bus to Vector6/1
  Bus Selector9/1 -> Bus to Vector4/1
  [mu] -> Vehicle Body 3DOF External Longitudinal Wheels/5(Friction)
  Longitudinal Wheels 4DOF/2(RearAxlF) -> Vehicle Body 3DOF External Longitudinal Wheels/3("FwR ")
  Bus to Vector4/1 -> Subsystem4/5(pqr)  "pqr"
  Vehicle Body 3DOF External Longitudinal Wheels/3(" YWheel") -> Subsystem4/14(YWheel)  "YWheel"
  Vector Concatenate/1 -> Longitudinal Wheels 4DOF/4(Gnd), [Ground]
  Bus to Vector/1 -> Subsystem4/2(CgXYZ)  "CgXYZ"
  AxlTrq/1 -> Longitudinal Wheels 4DOF/2(AxlTrq)
  Vehicle Body 3DOF External Longitudinal Wheels/1(" Info") -> Bus Selector13/1, Bus Selector11/1, Bus Selector10/1, Longitudinal Wheels 4DOF/6(VehFdbk), Bus Selector8/1, Bus Selector12/1, Bus Selector7/1, Bus Selector9/1, Bus Selector6/1, Bus Selector5/1
  [Ground] -> For 3D Visualization/3(GroundZ)
  Bus to Vector1/1 -> Subsystem4/3(CgXYZdot)  "CgXYZdot"
  Bus to Vector3/1 -> For 3D Visualization/1(angleIn)
  Longitudinal Wheels 4DOF/5(Alpha) -> Subsystem4/12(Alpha)  "Alpha"
  Vector Concatenate1/1 -> Longitudinal Wheels 4DOF/5(lam_mu), [mu]
  Bus Selector6/1 -> Bus to Vector1/1
  Brake Pressure/1(BrakePrs) -> Longitudinal Wheels 4DOF/3(BrkPrs)
  Vehicle Body 3DOF External Longitudinal Wheels/2(" XWheel") -> Subsystem4/13(XWheel)  "XWheel"
  Longitudinal Wheels 4DOF/4(Kappa) -> Subsystem4/11(Kappa)  "Kappa"
  Steering/1(WhlAng) -> Longitudinal Wheels 4DOF/1(WhlAng), Vehicle Body 3DOF External Longitudinal Wheels/1(WhlAng)
  Longitudinal Wheels 4DOF/6(zAxle) -> Subsystem4/15(dzWheel)  "dzWheel"
  Bus Selector7/1 -> Bus to Vector2/1
  Longitudinal Wheels 4DOF/3(Omega) -> Subsystem4/10(Omega)  "Omega"
  Bus Creator/1 -> RototestInput/1
  RototestDummy/1(CarTrqT2W) -> Bus Creator/1
  RototestDummy/2(AxleTrq) -> Bus Creator/2
  RototestDummy/3(BrakePressed_flag) -> Bus Creator/3
  RototestDummy/4(<VehSpd>) -> Bus Creator/4
  RototestDummy/5(<Fx>) -> Bus Creator/5

== system CM13_2024a_MachE_for_UA_HIL/Vehicle Under Test3/Vehicle/Vehicle Dynamics/Vehicle Longitudinal ==
  Env : Inport
  SupvsryCtrl : Inport  Port=2
  AxlTrq : Inport  Port=3
  Brake Pressure : Subsystem
  Bus Creator : BusCreator  Inputs=5
  Bus Selector1 : BusSelector  OutputSignals=BrkCmd
  Bus Selector2 : BusSelector  OutputSignals=RoadGrade,WindVel,GndBus.z,GndBus.mu
  Bus Selector3 : BusSelector  OutputSignals=G_FL_z,G_FR_z,G_RL_z,G_RR_z
  Bus Selector4 : BusSelector  OutputSignals=mu_FL,mu_FR,mu_RL,mu_RR
  Constant : Constant  Value=0
  Longitudinal Wheels : Subsystem  AncestorBlock=LibWheels/Longitudinal Wheels and Brakes
  RototestDummy : Subsystem
  Selector : Selector  InputPortWidth=3  IndexOptions=Index vector (dialog)  Indices=1  OutputSizes=1
  Terminator : Terminator
  Terminator1 : Terminator
  Vector Concatenate : Concatenate  NumInputs=4
  Vector Concatenate1 : Concatenate  NumInputs=4
  Vector Concatenate2 : Concatenate  NumInputs=4
  Vehicle Body : Subsystem
  Whl : Outport
  Chassis : Outport  Port=2
  RototestInput : Outport  Port=3
  wires:
  Vehicle Body/1(Chassis) -> Chassis/1
  Longitudinal Wheels/1(Whl) -> Whl/1
  Bus Selector4/1 -> Vector Concatenate1/1  "<mu_FL>"
  Bus Selector2/4 -> Bus Selector4/1  "<mu>"
  Vector Concatenate1/1 -> Terminator1/1
  Brake Pressure/1(BrakePrs) -> Longitudinal Wheels/1(BrkPrs)
  Bus Selector4/2 -> Vector Concatenate1/2  "<mu_FR>"
  Bus Selector3/1 -> Vector Concatenate/1  "<G_FL_z>"
  Bus Selector3/4 -> Vector Concatenate/4  "<G_RR_z>"
  Bus Selector2/3 -> Bus Selector3/1  "<z>"
  Env/1 -> Bus Selector2/1
  Vector Concatenate/1 -> Terminator/1
  Bus Selector4/3 -> Vector Concatenate1/3  "<mu_RL>"
  Bus Selector3/2 -> Vector Concatenate/2  "<G_FR_z>"
  SupvsryCtrl/1 -> Bus Selector1/1
  Constant/1 -> Vector Concatenate2/4, Vector Concatenate2/3, Vector Concatenate2/2, Vector Concatenate2/1
  Bus Selector4/4 -> Vector Concatenate1/4  "<mu_RR>"
  Bus Selector1/1 -> Brake Pressure/1(BrkReq)  "<BrkCmd>"
  Bus Selector3/3 -> Vector Concatenate/3  "<G_RL_z>"
  AxlTrq/1 -> Longitudinal Wheels/2(AxleTorq)
  Bus Selector2/2 -> Selector/1  "<WindVel>"
  Bus Selector2/1 -> Vehicle Body/1(RoadGrade)  "<RoadGrade>"
  Selector/1 -> Vehicle Body/2(WindX)
  Bus Creator/1 -> RototestInput/1
  RototestDummy/5(<Fx>) -> Bus Creator/5
  RototestDummy/4(<VehSpd>) -> Bus Creator/4
  RototestDummy/3(BrakePressed_flag) -> Bus Creator/3
  RototestDummy/2(AxleTrq) -> Bus Creator/2
  RototestDummy/1(CarTrqT2W) -> Bus Creator/1
  connections:
  Longitudinal Wheels/RConn2 -- Vehicle Body/LConn2
  Vehicle Body/LConn1 -- Longitudinal Wheels/RConn1

== system CM13_2024a_MachE_for_UA_HIL/CarMaker/IPG Vehicle/AEB Flag/RTICANMM ControllerSetup/ModelClose ==

== system CM13_2024a_MachE_for_UA_HIL/CarMaker/IPG Vehicle/AEB Flag/RTICANMM MainBlock/ModelClose ==

== system CM13_2024a_MachE_for_UA_HIL/CarMaker/IPG Vehicle/AEB Flag/RTICANMM MainBlock/converter ==
  in_1 : Inport
  in_2 : Inport  Port=2
  in_3 : Inport  Port=3
  in_4 : Inport  Port=4
  in_5 : Inport  Port=5
  in_6 : Inport  Port=6
  in_7 : Inport  Port=7
  ACCDATA_2 : BusCreator  Inputs=1
  Battery_Traction_2_FD1 : BusCreator  Inputs=2
  Mux : BusCreator  Inputs=3
  PowertrainData_10 : BusCreator  Inputs=4
  out : Outport
  wires:
  in_1/1 -> ACCDATA_2/1  "CmbbBrkDecel_A_Rq"
  ACCDATA_2/1 -> Mux/1  "ACCDATA_2"
  in_2/1 -> Battery_Traction_2_FD1/1  "BattTrac_U2_Actl"
  Battery_Traction_2_FD1/1 -> Mux/2  "Battery_Traction_2_FD1"
  in_3/1 -> Battery_Traction_2_FD1/2  "BattTrac_I2_Actl"
  in_4/1 -> PowertrainData_10/1  "TrnRng_D_Rq"
  PowertrainData_10/1 -> Mux/3  "PowertrainData_10"
  in_5/1 -> PowertrainData_10/2  "TrnPrkSys_D_Actl"
  in_6/1 -> PowertrainData_10/3  "GearPos_D_Actl"
  in_7/1 -> PowertrainData_10/4  "GearLvr_D_ActlDrv"
  Mux/1 -> out/1

== system CM13_2024a_MachE_for_UA_HIL/CarMaker/IPG Vehicle/Actuation and Outputs/MOOG Brake Actuator/ CAN Settings ==
  " CAN diagnostic Counter" : Subsystem  mask{TimeOutDuration=0.1}
      mask prompts: TimeOutDuration "CAN Time Out Duration"
  Data Type Conversion1 : DataTypeConversion  SaturateOnIntegerOverflow=off  RndMeth=Floor
  Data Type Conversion3 : DataTypeConversion  SaturateOnIntegerOverflow=off  RndMeth=Floor
  "RPDO3 Enable " : Constant
  RPDO3 period : Constant  Value=0.001
  RPDO3\PDU Features\PDU Cyclic Timing Control\RPDO3 Timing Control Period [BrakeAct_Config\Simulated ECUs\CANOpen_MOOG_02\Controller\TX\PDUs] : dsmpblib/Data Outport  Priority=-10000
      settings: SourceProductName=dSPACE Model Interface Package for Simulink (MIPS)
  RPDO3\PDU Features\PDU Enable\RPDO3 Enable [BrakeAct_Config\Simulated ECUs\CANOpen_MOOG_02\Controller\TX\PDUs] : dsmpblib/Data Outport  Priority=-10000
      settings: SourceProductName=dSPACE Model Interface Package for Simulink (MIPS)
  TPDO3\PDU Features\PDU RX Status\TPDO3 Counter [BrakeAct_Config\Simulated ECUs\CANOpen_MOOG_02\Controller\RX\PDUs] : dsmpblib/Data Inport  Priority=10000
      settings: SourceProductName=dSPACE Model Interface Package for Simulink (MIPS)
  CAN_CommsOK_Flg : Outport
  wires:
  "RPDO3 Enable "/1 -> Data Type Conversion3/1
  Data Type Conversion3/1 -> RPDO3\PDU Features\PDU Enable\RPDO3 Enable [BrakeAct_Config\Simulated ECUs\CANOpen_MOOG_02\Controller\TX\PDUs]/1
  RPDO3 period/1 -> RPDO3\PDU Features\PDU Cyclic Timing Control\RPDO3 Timing Control Period [BrakeAct_Config\Simulated ECUs\CANOpen_MOOG_02\Controller\TX\PDUs]/1
  TPDO3\PDU Features\PDU RX Status\TPDO3 Counter [BrakeAct_Config\Simulated ECUs\CANOpen_MOOG_02\Controller\RX\PDUs]/1 -> Data Type Conversion1/1
  Data Type Conversion1/1 -> " CAN diagnostic Counter"/1(RX Counter)
  " CAN diagnostic Counter"/1(CommsOKFlag) -> CAN_CommsOK_Flg/1  "TPDO3_CommsOK_Flg"

== system CM13_2024a_MachE_for_UA_HIL/CarMaker/IPG Vehicle/Actuation and Outputs/MOOG Brake Actuator/MOOG Interface ==
  note: Note: On 11.12.2024
      | Dyno test shows brake force is weak, Min offset is too low.
      | The value for MachE is set as:
      | Max Stop offiset: -5500, Min Stop offset: +3500 (different from Paul's suggested value in yellow box)
      | We adjusted to meet the requirement of "brake lights coming on at 4% and off at 1%"
      | Max Stop offset: -3500, Min Stop offset: +4100
  note: RAV4
      | Min an Max stops need adjusting otherwise:
      | - brake lights come on at 13% (with ajustment, it comes on at 2-3%
      | - 100% pedal can cause the actuator to generate a fault (maybe over current)
      | Min Offset +5500
      | Max Offset -5500
      |
      | Mach-e
      | Min Offset +5500
      | Max Offset -3500
      | this results in brake lights coming on at 4% and off at 1%
      |
      | total travel needs to be more than 35000 for valid range,
      | otherwise, brake booster was most likely not active
  CAN_CommsOK_Flg : Inport
  TargetPosition [pct] : Inport  Port=2
  StatusWord in : Inport  Port=3
  ActualPosition_cnt in : Inport  Port=4
  Mode of operation in : Inport  Port=5
  ActuatorMinTravelForReady : Constant  Value=35000
  Bus Creator : BusCreator  Inputs=2
  Constant1 : Constant  Value=100
  Constant2 : Constant  Value=100
  Data Type Conversion : DataTypeConversion  SaturateOnIntegerOverflow=off  RndMeth=Floor
  Data Type Conversion1 : DataTypeConversion  SaturateOnIntegerOverflow=off  RndMeth=Floor
  Display{2..5} (4 alike) : Display
  Gain : Gain
  Gain1 : Gain
  Gain2 : Gain
  MOOG State Machine : Stateflow chart  TreatAsAtomicUnit=on
  Max Stop Adjustment : Subsystem  TreatAsAtomicUnit=on
  Memory : Memory  InheritSampleTime=on
  Memory1 : Memory  InheritSampleTime=on
  Memory2 : Memory  InheritSampleTime=on
  Min Stop Adjustment : Subsystem  TreatAsAtomicUnit=on
  MoogResetCmd : Constant  Value=0
  PositionLearningTrigger : Constant  Value=0
  Product : Product  Inputs=*/*
  Product1 : Product  Inputs=*/*
  Rising edge : Subsystem
  Rising edge1 : Subsystem
  Sum : Sum  Inputs=|+-
  Sum1 : Sum  Inputs=|++
  Sum2 : Sum  Inputs=|+-
  Terminator{1..4} (4 alike) : Terminator
  Commands : Outport
  ActualPosition [pct] : Outport  Port=2
  BrakeActuatorReady : Outport  Port=3
  wires:
  Sum1/1 -> MOOG State Machine/6(TargetPosition_cnt)  "TargetPosition_cnt"
  Bus Creator/1 -> Commands/1
  [MaxStop_cnt] -> Sum/1
  [MinStop_cnt] -> Sum/2
  MOOG State Machine/1(ControlWord) -> Bus Creator/1  "ControlWord"
  MOOG State Machine/3(Actuator_Ready) -> BrakeActuatorReady/1  "Actuator_Ready"
  MOOG State Machine/4(FaultCntr) -> Display2/1  "FaultCounter"
  Sum/1 -> Product1/2, Product/3
  TargetPosition [pct]/1 -> Terminator3/1, Product/1  "TargetPosition_pct"
  Constant2/1 -> Product/2
  Gain/1 -> Data Type Conversion1/1, Sum2/1
  Gain1/1 -> Terminator1/1  "Mode of operation"
  Product/1 -> Sum1/1
  [MinStop_cnt] -> Sum2/2
  Sum2/1 -> Product1/1
  Constant1/1 -> Product1/3
  Product1/1 -> ActualPosition [pct]/1, Terminator2/1  "ActualPosition_pct"
  StatusWord in/1 -> Data Type Conversion/1
  Data Type Conversion/1 -> MOOG State Machine/4(StatusWord)  "StatusWord"
  ActualPosition_cnt in/1 -> Gain/1
  Mode of operation in/1 -> Gain1/1
  MOOG State Machine/5(MoogSMState) -> Display3/1  "MoogSMState"
  MOOG State Machine/6(InitComplete) -> Display4/1  "InitComplete"
  MOOG State Machine/7(MoogOpMode) -> Display5/1  "MoogOpMode"
  MOOG State Machine/10(MinStop) -> Memory1/1  "MinStop"
  MOOG State Machine/9(MaxStop) -> Memory/1  "MaxStop"
  MOOG State Machine/8(LearningComplete) -> Memory2/1  "LearningComplete"
  MOOG State Machine/2(PositionCmd) -> Gain2/1
  Gain2/1 -> Terminator4/1, Bus Creator/2  "TargetPositionFinal_cnt"
  Data Type Conversion1/1 -> MOOG State Machine/5(ActualPosition_cnt)  "ActualPosition_cnt"
  MoogResetCmd/1 -> Rising edge/1(In)
  Rising edge/1(Out) -> MOOG State Machine/2(ResetCmd)
  PositionLearningTrigger/1 -> Rising edge1/1(In)
  Rising edge1/1(Out) -> MOOG State Machine/3(PositionLearningTrigger)
  Max Stop Adjustment/1(Out1) -> [MaxStop_cnt]  "MaxStop_cnt"
  Min Stop Adjustment/1(Out1) -> [MinStop_cnt]  "MinStop_cnt"
  [MinStop_cnt] -> Sum1/2
  Memory/1 -> Max Stop Adjustment/1(In1)
  Memory1/1 -> Min Stop Adjustment/1(In1)
  Memory2/1 -> Max Stop Adjustment/Enable, Min Stop Adjustment/Enable
  CAN_CommsOK_Flg/1 -> MOOG State Machine/1(CAN_CommsOK_Flg)
  ActuatorMinTravelForReady/1 -> MOOG State Machine/7(ActuatorMinTravelForReady)

== system CM13_2024a_MachE_for_UA_HIL/CarMaker/IPG Vehicle/CarAndTrailer/CarAndTrailerUpd/CreateBus Brake.IF.In ==
  In : Inport
  BusCreator : BusCreator  Inputs=9
  Demux : Demux  Outputs=9
      settings: DisplayOption=none
  Out : Outport  VectorParamsAs1DForOutWhenUnconnected=off
  wires:
  Demux/9 -> BusCreator/9  "Brake IF Trq_Reg RR"
  Demux/8 -> BusCreator/8  "Brake IF Trq_Reg RL"
  Demux/7 -> BusCreator/7  "Brake IF Trq_Reg FR"
  Demux/6 -> BusCreator/6  "Brake IF Trq_Reg FL"
  Demux/5 -> BusCreator/5  "Brake IF Trq_Reg_max RR"
  Demux/4 -> BusCreator/4  "Brake IF Trq_Reg_max RL"
  Demux/3 -> BusCreator/3  "Brake IF Trq_Reg_max FR"
  Demux/2 -> BusCreator/2  "Brake IF Trq_Reg_max FL"
  Demux/1 -> BusCreator/1  "Brake IF T_env"
  BusCreator/1 -> Out/1
  In/1 -> Demux/1
